simulink model "state_fb_model_v2"  (R2019a)
settings: Solver=ode4  StartTime=0.0  StopTime=endtime  FixedStep=0.001  RelTol=1e-3
values from neighbouring files (symbols this model uses):
  bike_m = bike    [Untitled2.m]
undefined symbols (not defined in the file or in its folder): K
settings Model: Creator=chris  LastModifiedBy=chris

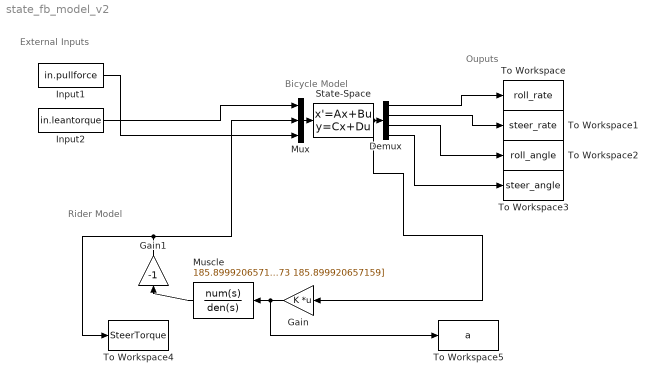
== system state_fb_model_v2 ==
  note: Bicycle Model
  note: External Inputs
  note: Rider Model
  note: Ouputs
  Demux : Demux
  Gain : Gain  Gain=K  Multiplication=Matrix(K*u) (u vector)
  Gain1 : Gain  Gain=-1
  Input1 : FromWorkspace  VariableName=in.pullforce  SampleTime=0
  Input2 : FromWorkspace  VariableName=in.leantorque  SampleTime=0
  Muscle : TransferFcn  Numerator=185.899920657159  Denominator=[1 19.2821119516073 185.899920657159]
  Mux : Mux  Inputs=3
  State-Space : StateSpace  A=bike_m.A  B=bike_m.B  C=bike_m.C  D=bike_m.D  InitialCondition=0
  To Workspace : ToWorkspace  VariableName=roll_rate  SampleTime=-1
  To Workspace1 : ToWorkspace  VariableName=steer_rate  SampleTime=-1
  To Workspace2 : ToWorkspace  VariableName=roll_angle  SampleTime=-1
  To Workspace3 : ToWorkspace  VariableName=steer_angle  SampleTime=-1
  To Workspace4 : ToWorkspace  VariableName=SteerTorque  SampleTime=-1
  To Workspace5 : ToWorkspace  VariableName=a  SampleTime=-1
  wires:
  Gain/1 -> To Workspace5/1, Muscle/1
  Gain1/1 -> Mux/2, To Workspace4/1
  Input1/1 -> Mux/3
  Mux/1 -> State-Space/1
  Demux/1 -> To Workspace/1
  Demux/2 -> To Workspace1/1
  Demux/3 -> To Workspace2/1
  Input2/1 -> Mux/1
  Muscle/1 -> Gain1/1
  Demux/4 -> To Workspace3/1
  State-Space/1 -> Gain/1, Demux/1
